simulink model "Modele_pendule_b"  (R2020b)
settings: Solver=VariableStepAuto  StartTime=0.0  StopTime=20  RelTol=1e-3
undefined symbols (not defined in the file or in its folder): Kx, now, x_0
settings Model: Creator=georgesghazi  LastModifiedBy=georgesghazi

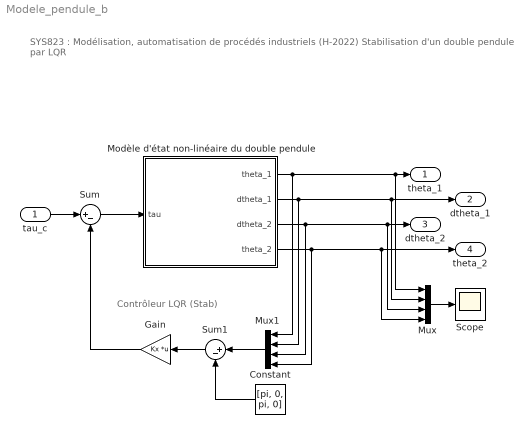
== system Modele_pendule_b ==
  note: Contrôleur LQR (Stab)
  note: SYS823 : Modélisation, automatisation de procédés industriels (H-2022)
      |
      | Stabilisation d'un double pendule par LQR
  tau_c : Inport
  Constant : Constant  Value=[pi, 0, pi, 0]
  Gain : Gain  Gain=Kx  Multiplication=Matrix(K*u) (u vector)
  Modèle d'état non-linéaire du double pendule : Subsystem
  Mux : Mux
  Mux1 : Mux
  Scope : Scope
  Sum : Sum  Inputs=|+-
  Sum1 : Sum  Inputs=|+-
  theta_1 : Outport
  dtheta_1 : Outport  Port=2
  dtheta_2 : Outport  Port=3
  theta_2 : Outport  Port=4
  wires:
  Mux/1 -> Scope/1
  Modèle d'état non-linéaire du double pendule/1(theta_1) -> Mux1/1, Mux/1, theta_1/1
  Modèle d'état non-linéaire du double pendule/2(dtheta_1) -> Mux1/2, Mux/2, dtheta_1/1
  Modèle d'état non-linéaire du double pendule/3(dtheta_2) -> Mux1/3, Mux/3, dtheta_2/1
  Modèle d'état non-linéaire du double pendule/4(theta_2) -> Mux1/4, theta_2/1, Mux/4
  Sum/1 -> Modèle d'état non-linéaire du double pendule/1(tau)
  Sum1/1 -> Gain/1
  Mux1/1 -> Sum1/1
  Constant/1 -> Sum1/2
  tau_c/1 -> Sum/1
  Gain/1 -> Sum/2

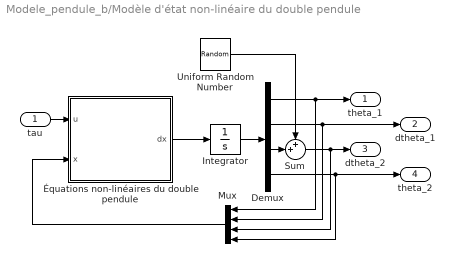
== system Modele_pendule_b/Modèle d'état non-linéaire du double pendule ==
  tau : Inport
  Demux : Demux
  Integrator : Integrator  InitialCondition=x_0
  Mux : Mux
  Sum : Sum  Inputs=++|
  Uniform Random Number : UniformRandomNumber  Minimum=-15*pi/180  Maximum=+15*pi/180  Seed=round(now)  SampleTime=5
  Équations non-linéaires du double pendule : MATLAB Function  TreatAsAtomicUnit=on
  theta_1 : Outport
  dtheta_1 : Outport  Port=2
  dtheta_2 : Outport  Port=3
  theta_2 : Outport  Port=4
  wires:
  Équations non-linéaires du double pendule/1(dx) -> Integrator/1
  Integrator/1 -> Demux/1
  tau/1 -> Équations non-linéaires du double pendule/1(u)
  Demux/2 -> Mux/2, dtheta_1/1
  Demux/4 -> Mux/4, theta_2/1
  Demux/1 -> theta_1/1, Mux/1
  Mux/1 -> Équations non-linéaires du double pendule/2(x)
  Demux/3 -> Sum/2
  Sum/1 -> Mux/3, dtheta_2/1
  Uniform Random Number/1 -> Sum/1

== matlab function Modele_pendule_b/Modèle d'état non-linéaire du double pendule/Équations non-linéaires du double pendule ==
  data: u input; dx output; x input
function dx = fcn(u, x)
% Déclaration des constantes 
m_1 = 1; m_2 = 1;
l_1 = 2; l_2 = 2;
g_0 = 9.81;

% Calcul de la dérivée du vecteur d'état
dx = zeros(size(x));

dx(1) = x(2);
dx(2) = -(l_1*l_2*m_2*sin(x(1) - x(3))*x(4)^2 - u - l_1*m_2*cos(x(1) - x(3))*(g_0*sin(x(3)) - ...
    l_1*x(2)^2*sin(x(1) - x(3))) + g_0*l_1*m_1*sin(x(1)) + g_0*l_1*m_2*sin(x(1)))/(l_1^2*m_1 + l_1^2*m_2);
dx(3) = x(4);
dx(4) = (l_1*sin(x(1) - x(3))*x(2)^2 - g_0*sin(x(3)) + (l_1*cos(x(1) - x(3))*...
    (l_1*l_2*m_2*sin(x(1) - x(3))*x(4)^2 - u + g_0*l_1*m_1*sin(x(1)) + ...
    g_0*l_1*m_2*sin(x(1))))/(l_1^2*m_1 + l_1^2*m_2))/l_2;
